simulink model "z3_1"  (R2017b)
settings: Solver=FixedStepDiscrete  StartTime=0.0  StopTime=0  RelTol=1e-3
undefined symbols (not defined in the file or in its folder): W
libraries: CPOiS_SourcesSinks x8, CPOiS_LinearTransforms x6, CPOiS_Filters x4, CPOiS_DataManipulation_DataTypeConversion x4
settings Model: Creator=alis  LastModifiedBy=alis

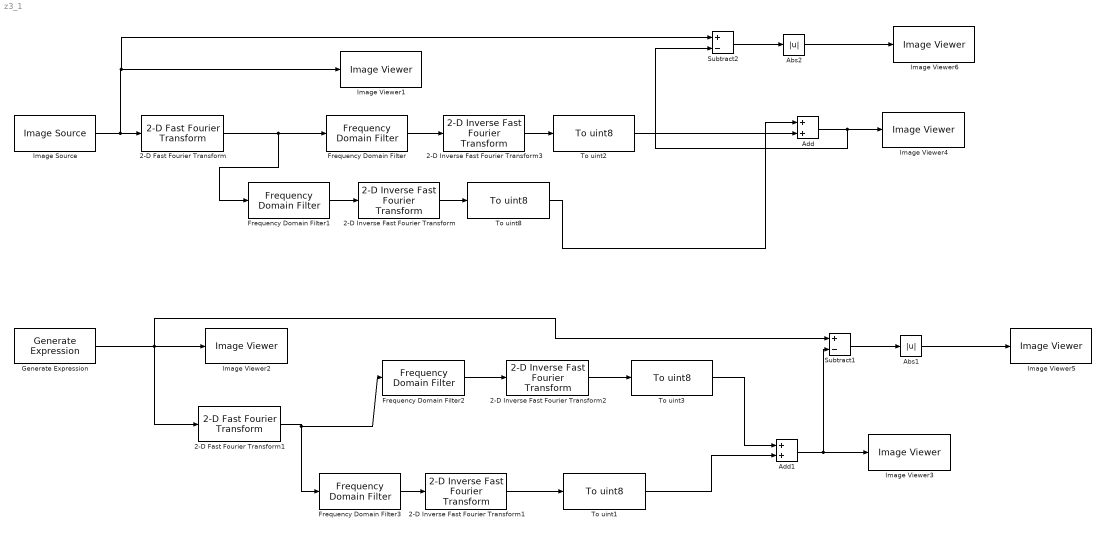
== system z3_1 ==
  2-D Fast Fourier Transform : CPOiS_LinearTransforms/2-D Fast Fourier Transform
      settings: SourceProductName=CPOiS - Digital image and signal processing
  2-D Fast Fourier Transform1 : CPOiS_LinearTransforms/2-D Fast Fourier Transform
      settings: SourceProductName=CPOiS - Digital image and signal processing
  2-D Inverse Fast Fourier Transform{,1..3} (4 alike) : CPOiS_LinearTransforms/2-D Inverse Fast  Fourier Transform
      settings: SourceProductName=CPOiS - Digital image and signal processing
  Abs1 : Abs
  Abs2 : Abs
  Add : Sum
  Add1 : Sum
  Frequency Domain Filter : CPOiS_Filters/Frequency Domain Filter  filtertype=Low-pass Filter  radius=10
      settings: SourceProductName=CPOiS - Digital image and signal processing
  Frequency Domain Filter1 : CPOiS_Filters/Frequency Domain Filter  filtertype=High-pass Filter  radius=10
      settings: SourceProductName=CPOiS - Digital image and signal processing
  Frequency Domain Filter2 : CPOiS_Filters/Frequency Domain Filter  filtertype=Low-pass Filter  radius=10
      settings: SourceProductName=CPOiS - Digital image and signal processing
  Frequency Domain Filter3 : CPOiS_Filters/Frequency Domain Filter  filtertype=High-pass Filter  radius=10
      settings: SourceProductName=CPOiS - Digital image and signal processing
  Generate Expression : CPOiS_SourcesSinks/Generate Expression  Width=256  Height=256  Expression=128.*(sin(W)+1)
      settings: SourceProductName=CPOiS - Digital image and signal processing
  Image Source : CPOiS_SourcesSinks/Image Source  FileSelection=marine.png
      settings: SourceProductName=CPOiS - Digital image and signal processing
  Image Viewer{1..6} (6 alike) : CPOiS_SourcesSinks/Image Viewer
      settings: SourceProductName=CPOiS - Digital image and signal processing
  Subtract1 : Sum  Inputs=+-
  Subtract2 : Sum  Inputs=+-
  To uint{1..3,8} (4 alike) : CPOiS_DataManipulation_DataTypeConversion/To uint8
      settings: SourceProductName=CPOiS - Digital image and signal processing
  wires:
  2-D Fast Fourier Transform1/1 -> Frequency Domain Filter2/1, Frequency Domain Filter3/1
  Add/1 -> Subtract2/2, Image Viewer4/1
  2-D Inverse Fast Fourier Transform/1 -> To uint8/1
  Image Source/1 -> Subtract2/1, Image Viewer1/1, 2-D Fast Fourier Transform/1
  Generate Expression/1 -> Subtract1/1, Image Viewer2/1, 2-D Fast Fourier Transform1/1
  Frequency Domain Filter/1 -> 2-D Inverse Fast Fourier Transform3/1
  To uint8/1 -> Add/1
  2-D Inverse Fast Fourier Transform1/1 -> To uint1/1
  2-D Fast Fourier Transform/1 -> Frequency Domain Filter1/1, Frequency Domain Filter/1
  Frequency Domain Filter1/1 -> 2-D Inverse Fast Fourier Transform/1
  To uint2/1 -> Add/2
  Subtract2/1 -> Abs2/1
  Abs2/1 -> Image Viewer6/1
  Frequency Domain Filter3/1 -> 2-D Inverse Fast Fourier Transform1/1
  Frequency Domain Filter2/1 -> 2-D Inverse Fast Fourier Transform2/1
  2-D Inverse Fast Fourier Transform3/1 -> To uint2/1
  2-D Inverse Fast Fourier Transform2/1 -> To uint3/1
  To uint1/1 -> Add1/2
  To uint3/1 -> Add1/1
  Add1/1 -> Subtract1/2, Image Viewer3/1
  Subtract1/1 -> Abs1/1
  Abs1/1 -> Image Viewer5/1
